simulink model "practical_class_3_2b_simulink"  (R2023b)
settings: Solver=VariableStepAuto  StartTime=0.0  StopTime=12  RelTol=1e-3
undefined symbols (not defined in the file): A, B, C, D
settings Model: Creator=klysm  LastModifiedBy=klysm

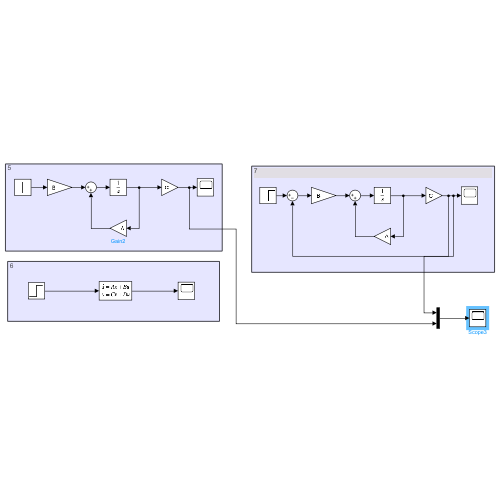
[thumbnail: Simulink's stored preview of the top-level diagram]
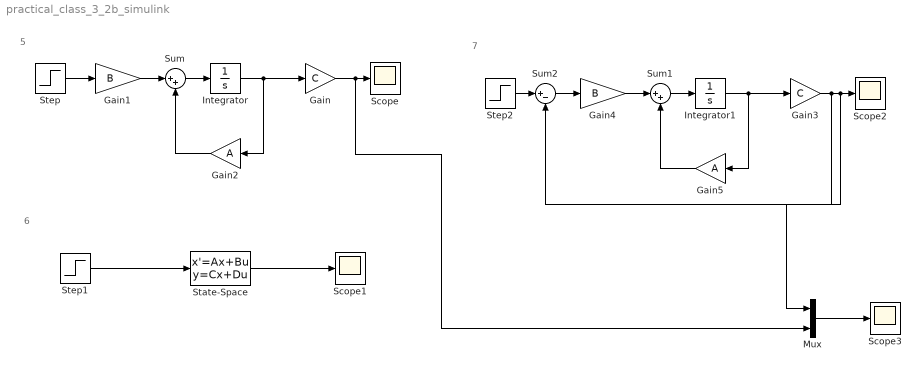
== system practical_class_3_2b_simulink ==
  note: 7
  note: 6
  note: 5
  Gain : Gain  Gain=C
  Gain1 : Gain  Gain=B
  Gain2 : Gain  Gain=A
  Gain3 : Gain  Gain=C
  Gain4 : Gain  Gain=B
  Gain5 : Gain  Gain=A
  Integrator : Integrator
  Integrator1 : Integrator
  Mux : Mux  Inputs=2
  Scope{,1..3} (4 alike) : Scope
  State-Space : StateSpace  A=A  B=B  C=C  D=D  InitialCondition=0
  Step : Step  Time=0  SampleTime=0
  Step1 : Step  Time=0  SampleTime=0
  Step2 : Step  Time=0  SampleTime=0
  Sum : Sum  Inputs=|++
  Sum1 : Sum  Inputs=|++
  Sum2 : Sum  Inputs=|+-
  wires:
  Integrator/1 -> Gain/1, Gain2/1
  Gain/1 -> Mux/2, Scope/1
  Sum/1 -> Integrator/1
  Gain1/1 -> Sum/1
  Step/1 -> Gain1/1
  Gain2/1 -> Sum/2
  State-Space/1 -> Scope1/1
  Step1/1 -> State-Space/1
  Gain5/1 -> Sum1/2
  Step2/1 -> Sum2/1
  Gain4/1 -> Sum1/1
  Sum1/1 -> Integrator1/1
  Gain3/1 -> Sum2/2, Mux/1, Scope2/1
  Integrator1/1 -> Gain5/1, Gain3/1
  Sum2/1 -> Gain4/1
  Mux/1 -> Scope3/1
